simulink model "process_lag_ports"  (R2018b)
settings: Solver=VariableStepAuto  StartTime=0.0  StopTime=10.0  RelTol=1e-3
libraries: simulink x1
settings Model: Creator=jh2044  LastModifiedBy=jh2044

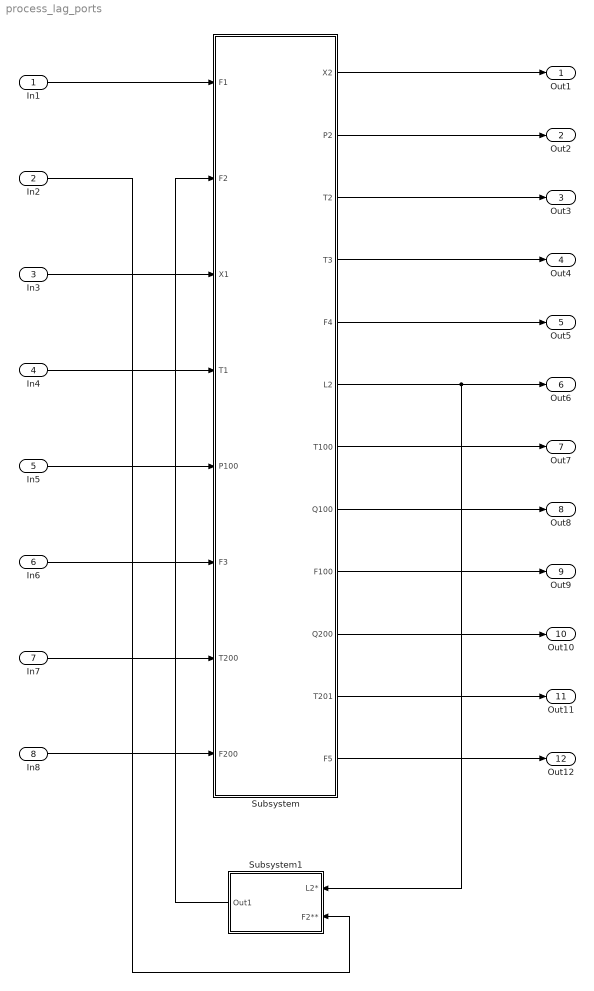
== system process_lag_ports ==
  In1 : Inport
  In2 : Inport  Port=2
  In3 : Inport  Port=3
  In4 : Inport  Port=4
  In5 : Inport  Port=5
  In6 : Inport  Port=6
  In7 : Inport  Port=7
  In8 : Inport  Port=8
  Subsystem : Subsystem
  Subsystem1 : Subsystem
  Out1 : Outport
  Out2 : Outport  Port=2
  Out3 : Outport  Port=3
  Out4 : Outport  Port=4
  Out5 : Outport  Port=5
  Out6 : Outport  Port=6
  Out7 : Outport  Port=7
  Out8 : Outport  Port=8
  Out9 : Outport  Port=9
  Out10 : Outport  Port=10
  Out11 : Outport  Port=11
  Out12 : Outport  Port=12
  wires:
  Subsystem/5(F4) -> Out5/1
  Subsystem/1(X2) -> Out1/1
  In5/1 -> Subsystem/5(P100)
  Subsystem/11(T201) -> Out11/1
  Subsystem/12(F5) -> Out12/1
  Subsystem/10(Q200) -> Out10/1
  Subsystem/9(F100) -> Out9/1
  Subsystem1/1(Out1) -> Subsystem/2(F2)
  In6/1 -> Subsystem/6(F3)
  In3/1 -> Subsystem/3(X1)
  Subsystem/2(P2) -> Out2/1
  Subsystem/4(T3) -> Out4/1
  Subsystem/8(Q100) -> Out8/1
  In8/1 -> Subsystem/8(F200)
  In4/1 -> Subsystem/4(T1)
  In1/1 -> Subsystem/1(F1)
  In2/1 -> Subsystem1/2(F2**)
  Subsystem/7(T100) -> Out7/1
  Subsystem/3(T2) -> Out3/1
  Subsystem/6(L2) -> Out6/1, Subsystem1/1(L2*)
  In7/1 -> Subsystem/7(T200)

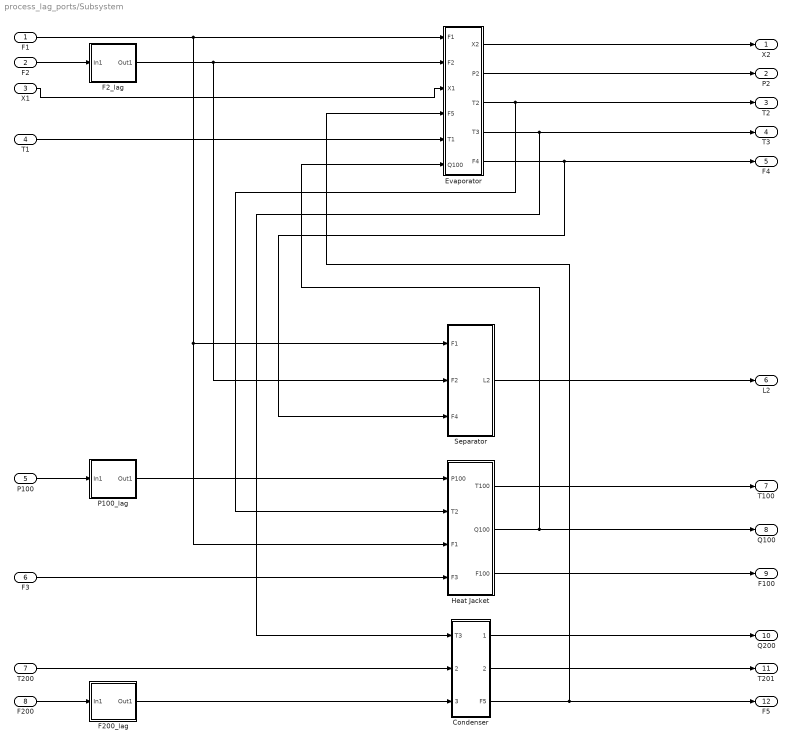
== system process_lag_ports/Subsystem ==
  F1 : Inport
  F2 : Inport  Port=2
  X1 : Inport  Port=3
  T1 : Inport  Port=4
  P100 : Inport  Port=5
  F3 : Inport  Port=6
  T200 : Inport  Port=7
  F200 : Inport  Port=8
  Condenser : Subsystem
  Evaporator : Subsystem
  F200_lag : Subsystem
  F2_lag : Subsystem
  Heat Jacket : Subsystem
  P100_lag : Subsystem
  Separator : Subsystem
  X2 : Outport
  P2 : Outport  Port=2
  T2 : Outport  Port=3
  T3 : Outport  Port=4
  F4 : Outport  Port=5
  L2 : Outport  Port=6
  T100 : Outport  Port=7
  Q100 : Outport  Port=8
  F100 : Outport  Port=9
  Q200 : Outport  Port=10
  T201 : Outport  Port=11
  F5 : Outport  Port=12
  wires:
  F200/1 -> F200_lag/1(In1)
  T1/1 -> Evaporator/5(T1)
  F1/1 -> Evaporator/1("F1 "), Separator/1(F1), Heat Jacket/3(F1)
  Heat Jacket/2(Q100) -> Q100/1, Evaporator/6(Q100)
  Evaporator/2(P2) -> P2/1
  Evaporator/5(F4) -> F4/1, Separator/3(F4)
  F2_lag/1(Out1) -> Separator/2("F2 "), Evaporator/2(F2)
  Condenser/1(Q200) -> Q200/1
  Condenser/3(F5) -> F5/1, Evaporator/4("F5 ")
  X1/1 -> Evaporator/3(X1)
  P100_lag/1(Out1) -> Heat Jacket/1(P100)
  Evaporator/3(T2) -> T2/1, Heat Jacket/2(T2)
  F3/1 -> Heat Jacket/4(F3)
  P100/1 -> P100_lag/1(In1)
  Condenser/2(T201) -> T201/1
  Heat Jacket/1(T100) -> T100/1
  Separator/1(L2) -> L2/1
  F2/1 -> F2_lag/1(In1)
  Heat Jacket/3(F100) -> F100/1
  Evaporator/4(T3) -> T3/1, Condenser/1(T3)
  T200/1 -> Condenser/2(T200)
  Evaporator/1("X2 ") -> X2/1
  F200_lag/1(Out1) -> Condenser/3(F200)

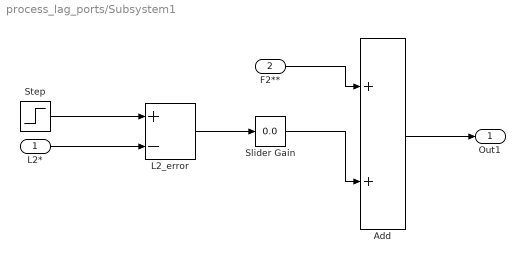
== system process_lag_ports/Subsystem1 ==
  L2* : Inport
  F2** : Inport  Port=2
  Add : Sum
  L2_error : Sum  Inputs=+-
  Slider Gain : simulink/Math Operations/Slider Gain  gain=0.0  low=-70  high=0
  Step : Step  Time=500  Before=1  SampleTime=0
  Out1 : Outport
  wires:
  Step/1 -> L2_error/1
  F2**/1 -> Add/1
  L2*/1 -> L2_error/2
  L2_error/1 -> Slider Gain/1
  Slider Gain/1 -> Add/2
  Add/1 -> Out1/1

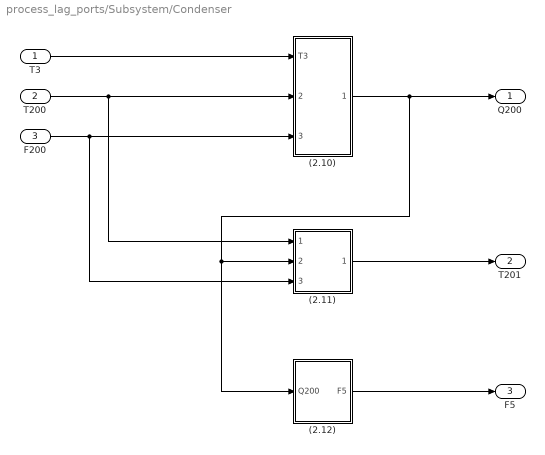
== system process_lag_ports/Subsystem/Condenser ==
  T3 : Inport
  T200 : Inport  Port=2
  F200 : Inport  Port=3
  (2.10) : Subsystem
  (2.11) : Subsystem
  (2.12) : Subsystem
  Q200 : Outport
  T201 : Outport  Port=2
  F5 : Outport  Port=3
  wires:
  (2.12)/1(F5) -> F5/1
  T200/1 -> (2.10)/2(T200), (2.11)/1(T200)
  T3/1 -> (2.10)/1(T3)
  F200/1 -> (2.11)/3(F200), (2.10)/3(F200)
  (2.10)/1(Q200) -> Q200/1, (2.12)/1(Q200), (2.11)/2(Q200)
  (2.11)/1(T201) -> T201/1

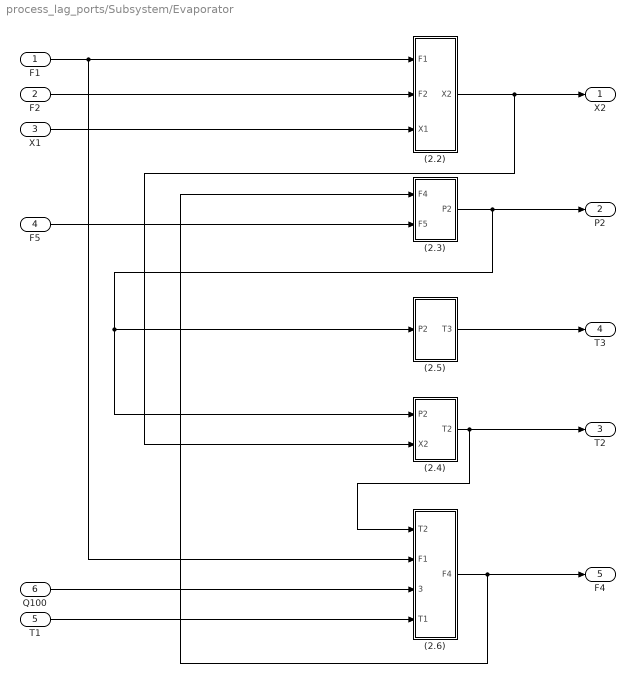
== system process_lag_ports/Subsystem/Evaporator ==
  "F1 " : Inport
  F2 : Inport  Port=2
  X1 : Inport  Port=3
  "F5 " : Inport  Port=4
  T1 : Inport  Port=5
  Q100 : Inport  Port=6
  (2.2) : Subsystem
  "(2.3) " : Subsystem
  (2.4) : Subsystem
  (2.5) : Subsystem
  (2.6) : Subsystem
  "X2 " : Outport
  P2 : Outport  Port=2
  T2 : Outport  Port=3
  T3 : Outport  Port=4
  F4 : Outport  Port=5
  wires:
  (2.2)/1("X2 ") -> "X2 "/1, (2.4)/2(X2)
  "F1 "/1 -> (2.6)/2(F1), (2.2)/1(F1)
  T1/1 -> (2.6)/4(T1)
  "(2.3) "/1(P2) -> P2/1, (2.4)/1(P2), (2.5)/1(P2)
  F2/1 -> (2.2)/2(F2)
  "F5 "/1 -> "(2.3) "/2("F5 ")
  (2.6)/1(F4) -> F4/1, "(2.3) "/1(F4)
  (2.4)/1(T2) -> T2/1, (2.6)/1(T2)
  X1/1 -> (2.2)/3(X1)
  Q100/1 -> (2.6)/3(Q100)
  (2.5)/1(T3) -> T3/1

== system process_lag_ports/Subsystem/F200_lag ==
  In1 : Inport
  1/T : Gain  Gain=1/1.2
  Integrator : Integrator  InitialCondition=208
  Sum : Sum  Inputs=|+-
  Out1 : Outport
  wires:
  1/T/1 -> Integrator/1
  Integrator/1 -> Out1/1, Sum/2
  In1/1 -> Sum/1
  Sum/1 -> 1/T/1

== system process_lag_ports/Subsystem/F2_lag ==
  In1 : Inport
  1/T : Gain  Gain=1/1.2
  Integrator : Integrator  InitialCondition=2
  Sum : Sum  Inputs=|+-
  Out1 : Outport
  wires:
  1/T/1 -> Integrator/1
  Integrator/1 -> Out1/1, Sum/2
  In1/1 -> Sum/1
  Sum/1 -> 1/T/1

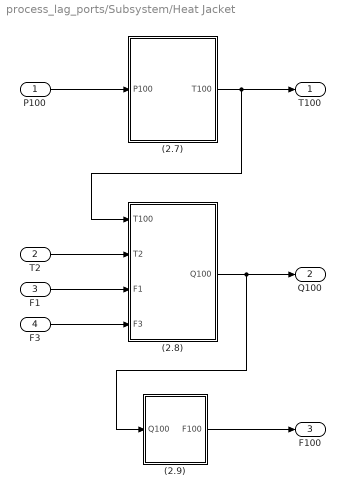
== system process_lag_ports/Subsystem/Heat Jacket ==
  P100 : Inport
  T2 : Inport  Port=2
  F1 : Inport  Port=3
  F3 : Inport  Port=4
  (2.7) : Subsystem
  (2.8) : Subsystem
  (2.9) : Subsystem
  T100 : Outport
  Q100 : Outport  Port=2
  F100 : Outport  Port=3
  wires:
  P100/1 -> (2.7)/1(P100)
  T2/1 -> (2.8)/2(T2)
  F3/1 -> (2.8)/4(F3)
  (2.8)/1(Q100) -> Q100/1, (2.9)/1(Q100)
  (2.9)/1(F100) -> F100/1
  F1/1 -> (2.8)/3(F1)
  (2.7)/1(T100) -> T100/1, (2.8)/1(T100)

== system process_lag_ports/Subsystem/P100_lag ==
  In1 : Inport
  1/T : Gain  Gain=1/1.2
  Integrator : Integrator  InitialCondition=194.7
  Sum : Sum  Inputs=|+-
  Out1 : Outport
  wires:
  1/T/1 -> Integrator/1
  Integrator/1 -> Out1/1, Sum/2
  In1/1 -> Sum/1
  Sum/1 -> 1/T/1

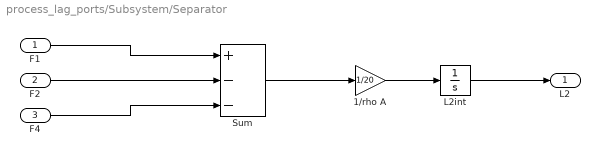
== system process_lag_ports/Subsystem/Separator ==
  F1 : Inport
  "F2 " : Inport  Port=2
  F4 : Inport  Port=3
  1/rho A : Gain  Gain=1/20
  L2int : Integrator
  Sum : Sum  Inputs=+--
  L2 : Outport
  wires:
  F4/1 -> Sum/3
  1/rho A/1 -> L2int/1
  "F2 "/1 -> Sum/2
  L2int/1 -> L2/1
  Sum/1 -> 1/rho A/1
  F1/1 -> Sum/1

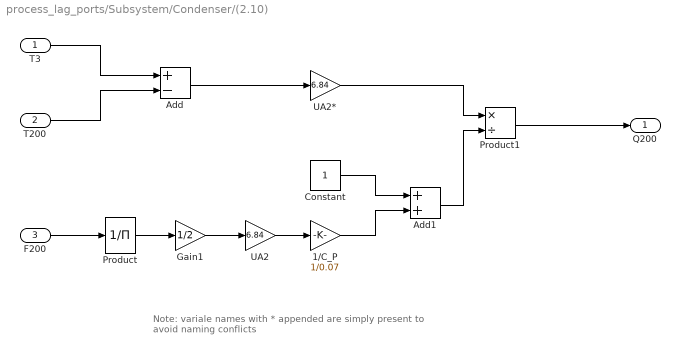
== system process_lag_ports/Subsystem/Condenser/(2.10) ==
  note: Note: variale names with * appended are simply present to avoid naming conflicts
  T3 : Inport
  T200 : Inport  Port=2
  F200 : Inport  Port=3
  1/C_P : Gain  Gain=1/0.07
  Add : Sum  Inputs=+-
  Add1 : Sum
  Constant : Constant
  Gain1 : Gain  Gain=1/2
  Product : Product  Inputs=/
  Product1 : Product  Inputs=*/
  UA2 : Gain  Gain=6.84
  UA2* : Gain  Gain=6.84
  Q200 : Outport
  wires:
  Product/1 -> Gain1/1
  F200/1 -> Product/1
  UA2*/1 -> Product1/1
  Gain1/1 -> UA2/1
  Product1/1 -> Q200/1
  1/C_P/1 -> Add1/2
  T3/1 -> Add/1
  T200/1 -> Add/2
  UA2/1 -> 1/C_P/1
  Constant/1 -> Add1/1
  Add/1 -> UA2*/1
  Add1/1 -> Product1/2

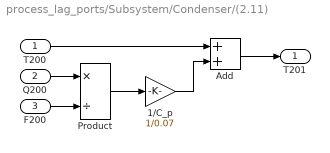
== system process_lag_ports/Subsystem/Condenser/(2.11) ==
  T200 : Inport
  Q200 : Inport  Port=2
  F200 : Inport  Port=3
  1/C_p : Gain  Gain=1/0.07
  Add : Sum
  Product : Product  Inputs=*/
  T201 : Outport
  wires:
  1/C_p/1 -> Add/2
  F200/1 -> Product/2
  T200/1 -> Add/1
  Product/1 -> 1/C_p/1
  Add/1 -> T201/1
  Q200/1 -> Product/1

== system process_lag_ports/Subsystem/Condenser/(2.12) ==
  Q200 : Inport
  "1/lambda " : Gain  Gain=1/38.5
  F5 : Outport
  wires:
  "1/lambda "/1 -> F5/1
  Q200/1 -> "1/lambda "/1

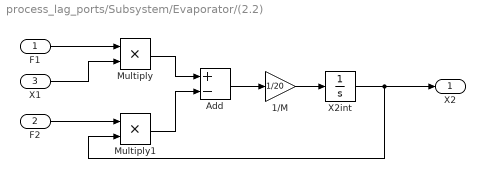
== system process_lag_ports/Subsystem/Evaporator/(2.2) ==
  F1 : Inport
  F2 : Inport  Port=2
  X1 : Inport  Port=3
  1/M : Gain  Gain=1/20
  Add : Sum  Inputs=+-
  Multiply : Product
  Multiply1 : Product
  X2int : Integrator
  "X2 " : Outport
  wires:
  Multiply1/1 -> Add/2
  Add/1 -> 1/M/1
  F1/1 -> Multiply/1
  X1/1 -> Multiply/2
  F2/1 -> Multiply1/1
  Multiply/1 -> Add/1
  X2int/1 -> "X2 "/1, Multiply1/2
  1/M/1 -> X2int/1

== system process_lag_ports/Subsystem/Evaporator/(2.3)  ==
  F4 : Inport
  "F5 " : Inport  Port=2
  1/C : Gain  Gain=1/4
  Add : Sum  Inputs=+-
  P2int : Integrator
  P2 : Outport
  wires:
  Add/1 -> 1/C/1
  F4/1 -> Add/1
  P2int/1 -> P2/1
  1/C/1 -> P2int/1
  "F5 "/1 -> Add/2

== system process_lag_ports/Subsystem/Evaporator/(2.4) ==
  P2 : Inport
  X2 : Inport  Port=2
  0.3126 : Gain  Gain=0.3126
  0.5616 : Gain  Gain=0.5616
  Add : Sum  Inputs=+++
  Constant : Constant  Value=48.43
  T2 : Outport
  wires:
  Constant/1 -> Add/3
  X2/1 -> 0.3126/1
  P2/1 -> 0.5616/1
  0.3126/1 -> Add/2
  0.5616/1 -> Add/1
  Add/1 -> T2/1

== system process_lag_ports/Subsystem/Evaporator/(2.5) ==
  P2 : Inport
  0.507 : Gain  Gain=0.507
  Add : Sum
  Constant : Constant  Value=55.0
  T3 : Outport
  wires:
  0.507/1 -> Add/1
  Add/1 -> T3/1
  Constant/1 -> Add/2
  P2/1 -> 0.507/1

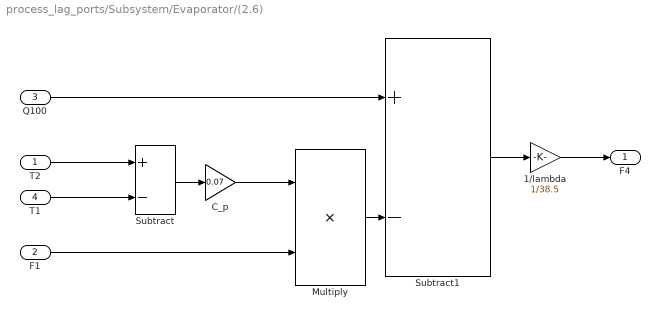
== system process_lag_ports/Subsystem/Evaporator/(2.6) ==
  T2 : Inport
  F1 : Inport  Port=2
  Q100 : Inport  Port=3
  T1 : Inport  Port=4
  1/lambda : Gain  Gain=1/38.5
  C_p : Gain  Gain=0.07
  Multiply : Product
  Subtract : Sum  Inputs=+-
  Subtract1 : Sum  Inputs=+-
  F4 : Outport
  wires:
  1/lambda/1 -> F4/1
  T2/1 -> Subtract/1
  Q100/1 -> Subtract1/1
  F1/1 -> Multiply/2
  Multiply/1 -> Subtract1/2
  Subtract1/1 -> 1/lambda/1
  C_p/1 -> Multiply/1
  T1/1 -> Subtract/2
  Subtract/1 -> C_p/1

== system process_lag_ports/Subsystem/Heat Jacket/(2.7) ==
  P100 : Inport
  Constant : Constant  Value=90.0
  Gain : Gain  Gain=0.1538
  Sum : Sum
  T100 : Outport
  wires:
  Gain/1 -> Sum/2
  P100/1 -> Gain/1
  Constant/1 -> Sum/1
  Sum/1 -> T100/1

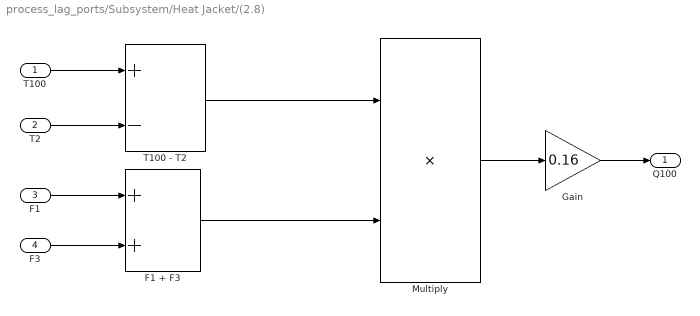
== system process_lag_ports/Subsystem/Heat Jacket/(2.8) ==
  T100 : Inport
  T2 : Inport  Port=2
  F1 : Inport  Port=3
  F3 : Inport  Port=4
  F1 + F3 : Sum
  Gain : Gain  Gain=0.16
  Multiply : Product
  T100 - T2 : Sum  Inputs=+-
  Q100 : Outport
  wires:
  Gain/1 -> Q100/1
  T2/1 -> T100 - T2/2
  T100/1 -> T100 - T2/1
  Multiply/1 -> Gain/1
  F1/1 -> F1 + F3/1
  T100 - T2/1 -> Multiply/1
  F1 + F3/1 -> Multiply/2
  F3/1 -> F1 + F3/2

== system process_lag_ports/Subsystem/Heat Jacket/(2.9) ==
  Q100 : Inport
  1/lambda_sigma : Gain  Gain=1/36.6
  F100 : Outport
  wires:
  1/lambda_sigma/1 -> F100/1
  Q100/1 -> 1/lambda_sigma/1
